simulink model "untitled"  (R2021b)
settings: Solver=VariableStepAuto  StartTime=0.0  StopTime=10.0  RelTol=1e-3
settings Model: Creator=user  LastModifiedBy=user

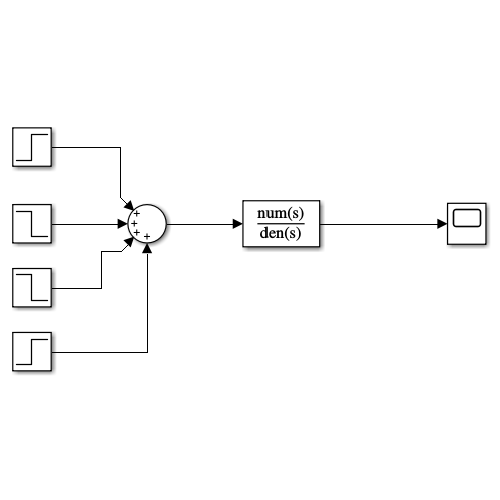
[thumbnail: Simulink's stored preview of the top-level diagram]
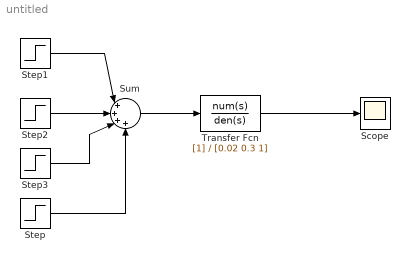
== system untitled ==
  Scope : Scope
  Step : Step  Time=8  SampleTime=0
  Step1 : Step  Time=2  SampleTime=0
  Step2 : Step  Time=4  After=-1  SampleTime=0
  Step3 : Step  Time=6  After=-1  SampleTime=0
  Sum : Sum  Inputs=|++++
  Transfer Fcn : TransferFcn  Denominator=[0.02 0.3 1]
  wires:
  Sum/1 -> Transfer Fcn/1
  Transfer Fcn/1 -> Scope/1
  Step1/1 -> Sum/1
  Step/1 -> Sum/4
  Step3/1 -> Sum/3
  Step2/1 -> Sum/2
